simulink model "Modelling2018"  (R2018b)
settings: Solver=VariableStepAuto  StartTime=0.0  StopTime=50  FixedStep=1/16000  RelTol=1e-3
values from neighbouring files (symbols this model uses):
  A = [0 1 0 0 ... (first row only)    [ControllerToProject.m]
  B = [0 0 ... (first row only)    [ControllerToProject.m]
  b = 1    [ControllerToProject.m]    (also in Parameters.m)
  C = [1 0 0 0 ... (first row only)    [ControllerToProject.m]
  g = 9.81    [ControllerToProject.m]    (also in Parameters.m = 9.82)
  l = 0.36022    [ControllerToProject.m]    (also in Parameters.m = 0.35)
  mc = 0.9+0.1    (= 1)    [ControllerToProject.m]    (also in Parameters.m = 0.9)
  mp = 0.08887    [ControllerToProject.m]    (also in Parameters.m = 0.1)
undefined symbols (not defined in the file or in its folder): F, Fi, sigbuilder_block
libraries: simulink x9, simulink_extras x3
settings Model: Creator=Emil  LastModifiedBy=Emil
settings SolverCC: AlgebraicLoopSolver=LineSearch
settings DataIOCC: ReturnWorkspaceOutputs=on

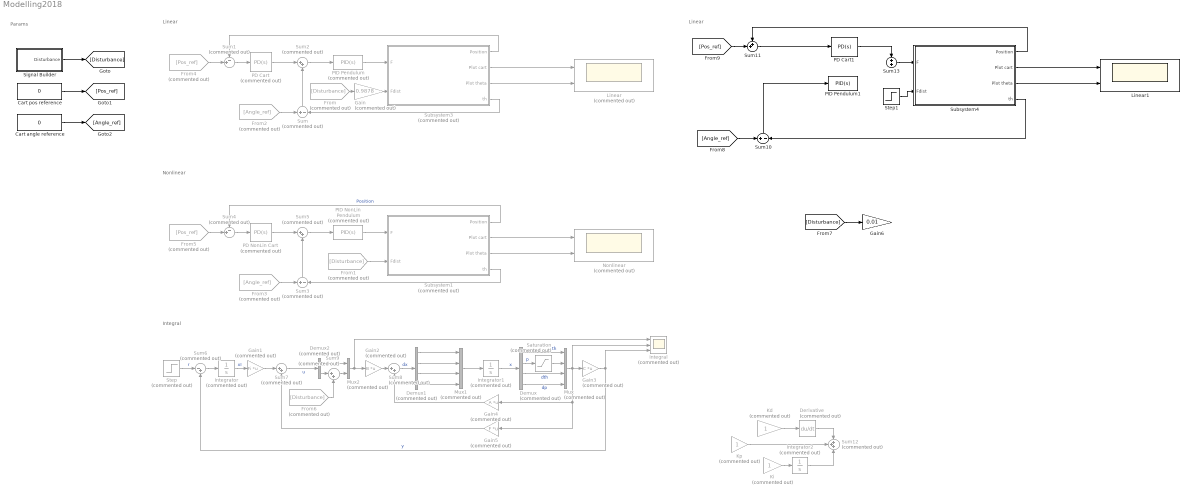
== system Modelling2018 ==
  note: Params
  note: Nonlinear
  note: Linear
  note: Integral
  note: Linear
  Cart angle reference : Constant  Value=0
  Cart pos reference : Constant  Value=0
  Demux : Demux  Commented=on
  Demux1 : Demux  Commented=on
  Demux2 : Demux  Commented=on  Outputs=2
  Derivative : Derivative  Commented=on
  From : From  Commented=on  GotoTag=Disturbance
  From1 : From  Commented=on  GotoTag=Disturbance
  From2 : From  Commented=on  GotoTag=Angle_ref
  From3 : From  Commented=on  GotoTag=Angle_ref
  From4 : From  Commented=on  GotoTag=Pos_ref
  From5 : From  Commented=on  GotoTag=Pos_ref
  From6 : From  Commented=on  GotoTag=Disturbance
  Gain : Gain  Commented=on  Gain=0.9878
  Gain1 : Gain  Commented=on  Gain=Fi  Multiplication=Matrix(K*u)
  Gain2 : Gain  Commented=on  Gain=B  Multiplication=Matrix(K*u)
  Gain3 : Gain  Commented=on  Gain=C  Multiplication=Matrix(K*u)
  Gain4 : Gain  Commented=on  Gain=A  Multiplication=Matrix(K*u)
  Gain5 : Gain  Commented=on  Gain=F  Multiplication=Matrix(K*u)
  Gain6 : Gain  Gain=0.01
  Integral : Scope  Commented=on  NumInputPorts=3
  Integrator : Integrator  Commented=on
  Integrator1 : Integrator  Commented=on
  Integrator2 : Integrator  Commented=on
  Kd : Gain  Commented=on
  Ki : Gain  Commented=on
  Kp : Gain  Commented=on
  Linear : Scope  Commented=on  NumInputPorts=2
  Linear1 : Scope  NumInputPorts=2
  Mux : Mux  Commented=on
  Mux1 : Mux  Commented=on
  Mux2 : Mux  Commented=on  Inputs=2
  Nonlinear : Scope  Commented=on  NumInputPorts=2
  PD Cart : simulink/Continuous/PID Controller  Commented=on  Controller=PD  Form=Ideal  TimeDomain=Continuous-time  SampleTime=-1  IntegratorMethod=Forward Euler  FilterMethod=Forward Euler  ControllerParametersSource=internal  P=1  I=0  D=0.017  UseFilter=on  N=100  TunerSelectOption=Transfer Function Based (PID Tuner App)  InitialConditionSource=internal  InitialConditionForIntegrator=0  InitialConditionForFilter=0  DifferentiatorICPrevScaledInput=0  ExternalReset=none  TrackingMode=off  Kt=1  LimitOutput=off  UpperSaturationLimit=inf  LowerSaturationLimit=-inf  LinearizeAsGain=on  AntiWindupMode=none  Kb=1  POutMin=[]  POutMax=[]  IOutMin=[]  IOutMax=[]  DOutMin=[]  DOutMax=[]  NOutMin=[]  NOutMax=[]  SumOutMin=[]  SumOutMax=[]  SaturationOutMin=[]  SaturationOutMax=[]  PParamMin=[]  PParamMax=[]  IParamMin=[]  IParamMax=[]  DParamMin=[]  DParamMax=[]  NParamMin=[]  NParamMax=[]  KbParamMin=[]  KbParamMax=[]  KtParamMin=[]  KtParamMax=[]  KbOutMin=[]  KbOutMax=[]  KtOutMin=[]  KtOutMax=[]  IntegratorOutMin=[]  IntegratorOutMax=[]  FilterOutMin=[]  FilterOutMax=[]  SumI1OutMin=[]  SumI1OutMax=[]  SumI2OutMin=[]  SumI2OutMax=[]  SumI3OutMin=[]  SumI3OutMax=[]  SumI4OutMin=[]  SumI4OutMax=[]  SumDOutMin=[]  SumDOutMax=[]  DifferentiatorOutMin=[]  DifferentiatorOutMax=[]  FilterDiffOutCoefMin=[]  FilterDiffOutCoefMax=[]  ReciprocalOutMin=[]  ReciprocalOutMax=[]  SumDenOutMin=[]  SumDenOutMax=[]  SumNumOutMin=[]  SumNumOutMax=[]  DivideOutMin=[]  DivideOutMax=[]  IntegratorContinuousStateAttributes=''  IntegratorStateMustResolveToSignalObject=off  IntegratorRTWStateStorageClass=Auto  FilterContinuousStateAttributes=''  FilterStateMustResolveToSignalObject=off  FilterRTWStateStorageClass=Auto  ParallelPVariant=Passthrough  IdealPVariant=InternalParameters  IVariant=Disabled  DVariant=InternalParameters  IntegratorVariant=Disabled  SatVariant=Disabled  AWVariant=Disabled  PCopyVariant=Disabled  TRVariant=Disabled  FdbkBlocksVariant=Forward  IdealPFdbkVariant=Disabled  SatFdbkVariant=Disabled  DerivativeFilterVariant=ContFilter  NVariant=InternalParameters  NCopyVariant=Disabled  FilterICVariant=InternalICsFilter  IntegratorICVariant=Disabled  ExternalResetVariant=Disabled  TRSumVariant=Passthrough  SumFdbkVariant=Disabled  SumVariant=Sum_PD
  PD Cart1 : simulink/Continuous/PID Controller  Controller=PD  Form=Parallel  TimeDomain=Continuous-time  SampleTime=-1  IntegratorMethod=Forward Euler  FilterMethod=Forward Euler  ControllerParametersSource=internal  P=1  I=1793804776.75566  D=0  UseFilter=on  N=100  TunerSelectOption=Transfer Function Based (PID Tuner App)  InitialConditionSource=internal  InitialConditionForIntegrator=0  InitialConditionForFilter=0  DifferentiatorICPrevScaledInput=0  ExternalReset=none  TrackingMode=off  Kt=1  LimitOutput=off  UpperSaturationLimit=50  LowerSaturationLimit=-50  LinearizeAsGain=on  AntiWindupMode=none  Kb=1  POutMin=[]  POutMax=[]  IOutMin=[]  IOutMax=[]  DOutMin=[]  DOutMax=[]  NOutMin=[]  NOutMax=[]  SumOutMin=[]  SumOutMax=[]  SaturationOutMin=[]  SaturationOutMax=[]  PParamMin=[]  PParamMax=[]  IParamMin=[]  IParamMax=[]  DParamMin=[]  DParamMax=[]  NParamMin=[]  NParamMax=[]  KbParamMin=[]  KbParamMax=[]  KtParamMin=[]  KtParamMax=[]  KbOutMin=[]  KbOutMax=[]  KtOutMin=[]  KtOutMax=[]  IntegratorOutMin=[]  IntegratorOutMax=[]  FilterOutMin=[]  FilterOutMax=[]  SumI1OutMin=[]  SumI1OutMax=[]  SumI2OutMin=[]  SumI2OutMax=[]  SumI3OutMin=[]  SumI3OutMax=[]  SumI4OutMin=[]  SumI4OutMax=[]  SumDOutMin=[]  SumDOutMax=[]  DifferentiatorOutMin=[]  DifferentiatorOutMax=[]  FilterDiffOutCoefMin=[]  FilterDiffOutCoefMax=[]  ReciprocalOutMin=[]  ReciprocalOutMax=[]  SumDenOutMin=[]  SumDenOutMax=[]  SumNumOutMin=[]  SumNumOutMax=[]  DivideOutMin=[]  DivideOutMax=[]  IntegratorContinuousStateAttributes=''  IntegratorStateMustResolveToSignalObject=off  IntegratorRTWStateStorageClass=Auto  FilterContinuousStateAttributes=''  FilterStateMustResolveToSignalObject=off  FilterRTWStateStorageClass=Auto  ParallelPVariant=InternalParameters  IdealPVariant=Disabled  IVariant=Disabled  DVariant=InternalParameters  IntegratorVariant=Disabled  SatVariant=Disabled  AWVariant=Disabled  PCopyVariant=Disabled  TRVariant=Disabled  FdbkBlocksVariant=Forward  IdealPFdbkVariant=Disabled  SatFdbkVariant=Disabled  DerivativeFilterVariant=ContFilter  NVariant=InternalParameters  NCopyVariant=Disabled  FilterICVariant=InternalICsFilter  IntegratorICVariant=Disabled  ExternalResetVariant=Disabled  TRSumVariant=Passthrough  SumFdbkVariant=Disabled  SumVariant=Sum_PD
  PD NonLin Cart : simulink/Continuous/PID Controller  Commented=on  Controller=PD  Form=Ideal  TimeDomain=Continuous-time  SampleTime=-1  IntegratorMethod=Forward Euler  FilterMethod=Forward Euler  ControllerParametersSource=internal  P=0.945  I=0  D=0.017  UseFilter=on  N=100  TunerSelectOption=Transfer Function Based (PID Tuner App)  InitialConditionSource=internal  InitialConditionForIntegrator=0  InitialConditionForFilter=0  DifferentiatorICPrevScaledInput=0  ExternalReset=none  TrackingMode=off  Kt=1  LimitOutput=off  UpperSaturationLimit=inf  LowerSaturationLimit=-inf  LinearizeAsGain=on  AntiWindupMode=none  Kb=1  POutMin=[]  POutMax=[]  IOutMin=[]  IOutMax=[]  DOutMin=[]  DOutMax=[]  NOutMin=[]  NOutMax=[]  SumOutMin=[]  SumOutMax=[]  SaturationOutMin=[]  SaturationOutMax=[]  PParamMin=[]  PParamMax=[]  IParamMin=[]  IParamMax=[]  DParamMin=[]  DParamMax=[]  NParamMin=[]  NParamMax=[]  KbParamMin=[]  KbParamMax=[]  KtParamMin=[]  KtParamMax=[]  KbOutMin=[]  KbOutMax=[]  KtOutMin=[]  KtOutMax=[]  IntegratorOutMin=[]  IntegratorOutMax=[]  FilterOutMin=[]  FilterOutMax=[]  SumI1OutMin=[]  SumI1OutMax=[]  SumI2OutMin=[]  SumI2OutMax=[]  SumI3OutMin=[]  SumI3OutMax=[]  SumI4OutMin=[]  SumI4OutMax=[]  SumDOutMin=[]  SumDOutMax=[]  DifferentiatorOutMin=[]  DifferentiatorOutMax=[]  FilterDiffOutCoefMin=[]  FilterDiffOutCoefMax=[]  ReciprocalOutMin=[]  ReciprocalOutMax=[]  SumDenOutMin=[]  SumDenOutMax=[]  SumNumOutMin=[]  SumNumOutMax=[]  DivideOutMin=[]  DivideOutMax=[]  IntegratorContinuousStateAttributes=''  IntegratorStateMustResolveToSignalObject=off  IntegratorRTWStateStorageClass=Auto  FilterContinuousStateAttributes=''  FilterStateMustResolveToSignalObject=off  FilterRTWStateStorageClass=Auto  ParallelPVariant=Passthrough  IdealPVariant=InternalParameters  IVariant=Disabled  DVariant=InternalParameters  IntegratorVariant=Disabled  SatVariant=Disabled  AWVariant=Disabled  PCopyVariant=Disabled  TRVariant=Disabled  FdbkBlocksVariant=Forward  IdealPFdbkVariant=Disabled  SatFdbkVariant=Disabled  DerivativeFilterVariant=ContFilter  NVariant=InternalParameters  NCopyVariant=Disabled  FilterICVariant=InternalICsFilter  IntegratorICVariant=Disabled  ExternalResetVariant=Disabled  TRSumVariant=Passthrough  SumFdbkVariant=Disabled  SumVariant=Sum_PD
  PID NonLin Pendulum : simulink/Continuous/PID Controller  Commented=on  Controller=PID  Form=Ideal  TimeDomain=Continuous-time  SampleTime=-1  IntegratorMethod=Forward Euler  FilterMethod=Forward Euler  ControllerParametersSource=internal  P=-500  I=55  D=5  UseFilter=on  N=500  TunerSelectOption=Transfer Function Based (PID Tuner App)  InitialConditionSource=internal  InitialConditionForIntegrator=0  InitialConditionForFilter=0  DifferentiatorICPrevScaledInput=0  ExternalReset=none  TrackingMode=off  Kt=1  LimitOutput=on  UpperSaturationLimit=50  LowerSaturationLimit=-50  LinearizeAsGain=on  AntiWindupMode=clamping  Kb=1  POutMin=[]  POutMax=[]  IOutMin=[]  IOutMax=[]  DOutMin=[]  DOutMax=[]  NOutMin=[]  NOutMax=[]  SumOutMin=[]  SumOutMax=[]  SaturationOutMin=[]  SaturationOutMax=[]  PParamMin=[]  PParamMax=[]  IParamMin=[]  IParamMax=[]  DParamMin=[]  DParamMax=[]  NParamMin=[]  NParamMax=[]  KbParamMin=[]  KbParamMax=[]  KtParamMin=[]  KtParamMax=[]  KbOutMin=[]  KbOutMax=[]  KtOutMin=[]  KtOutMax=[]  IntegratorOutMin=[]  IntegratorOutMax=[]  FilterOutMin=[]  FilterOutMax=[]  SumI1OutMin=[]  SumI1OutMax=[]  SumI2OutMin=[]  SumI2OutMax=[]  SumI3OutMin=[]  SumI3OutMax=[]  SumI4OutMin=[]  SumI4OutMax=[]  SumDOutMin=[]  SumDOutMax=[]  DifferentiatorOutMin=[]  DifferentiatorOutMax=[]  FilterDiffOutCoefMin=[]  FilterDiffOutCoefMax=[]  ReciprocalOutMin=[]  ReciprocalOutMax=[]  SumDenOutMin=[]  SumDenOutMax=[]  SumNumOutMin=[]  SumNumOutMax=[]  DivideOutMin=[]  DivideOutMax=[]  IntegratorContinuousStateAttributes=''  IntegratorStateMustResolveToSignalObject=off  IntegratorRTWStateStorageClass=Auto  FilterContinuousStateAttributes=''  FilterStateMustResolveToSignalObject=off  FilterRTWStateStorageClass=Auto  ParallelPVariant=Passthrough  IdealPVariant=InternalParameters  IVariant=InternalParameters  DVariant=InternalParameters  IntegratorVariant=Continuous  SatVariant=Enabled  AWVariant=ContClampingIdeal  PCopyVariant=InternalParamsIdeal  TRVariant=Disabled  FdbkBlocksVariant=Forward  IdealPFdbkVariant=Disabled  SatFdbkVariant=Disabled  DerivativeFilterVariant=ContFilter  NVariant=InternalParameters  NCopyVariant=Disabled  FilterICVariant=InternalICsFilter  IntegratorICVariant=InternalICs  ExternalResetVariant=Disabled  TRSumVariant=Passthrough  SumFdbkVariant=Disabled  SumVariant=Sum_PID
  PID Pendulum : simulink/Continuous/PID Controller  Commented=on  Controller=PID  Form=Ideal  TimeDomain=Continuous-time  SampleTime=-1  IntegratorMethod=Forward Euler  FilterMethod=Forward Euler  ControllerParametersSource=internal  P=-500  I=0.01  D=5  UseFilter=on  N=500  TunerSelectOption=Transfer Function Based (PID Tuner App)  InitialConditionSource=internal  InitialConditionForIntegrator=0  InitialConditionForFilter=0  DifferentiatorICPrevScaledInput=0  ExternalReset=none  TrackingMode=off  Kt=1  LimitOutput=on  UpperSaturationLimit=50  LowerSaturationLimit=-50  LinearizeAsGain=on  AntiWindupMode=clamping  Kb=1  POutMin=[]  POutMax=[]  IOutMin=[]  IOutMax=[]  DOutMin=[]  DOutMax=[]  NOutMin=[]  NOutMax=[]  SumOutMin=[]  SumOutMax=[]  SaturationOutMin=[]  SaturationOutMax=[]  PParamMin=[]  PParamMax=[]  IParamMin=[]  IParamMax=[]  DParamMin=[]  DParamMax=[]  NParamMin=[]  NParamMax=[]  KbParamMin=[]  KbParamMax=[]  KtParamMin=[]  KtParamMax=[]  KbOutMin=[]  KbOutMax=[]  KtOutMin=[]  KtOutMax=[]  IntegratorOutMin=[]  IntegratorOutMax=[]  FilterOutMin=[]  FilterOutMax=[]  SumI1OutMin=[]  SumI1OutMax=[]  SumI2OutMin=[]  SumI2OutMax=[]  SumI3OutMin=[]  SumI3OutMax=[]  SumI4OutMin=[]  SumI4OutMax=[]  SumDOutMin=[]  SumDOutMax=[]  DifferentiatorOutMin=[]  DifferentiatorOutMax=[]  FilterDiffOutCoefMin=[]  FilterDiffOutCoefMax=[]  ReciprocalOutMin=[]  ReciprocalOutMax=[]  SumDenOutMin=[]  SumDenOutMax=[]  SumNumOutMin=[]  SumNumOutMax=[]  DivideOutMin=[]  DivideOutMax=[]  IntegratorContinuousStateAttributes=''  IntegratorStateMustResolveToSignalObject=off  IntegratorRTWStateStorageClass=Auto  FilterContinuousStateAttributes=''  FilterStateMustResolveToSignalObject=off  FilterRTWStateStorageClass=Auto  ParallelPVariant=Passthrough  IdealPVariant=InternalParameters  IVariant=InternalParameters  DVariant=InternalParameters  IntegratorVariant=Continuous  SatVariant=Enabled  AWVariant=ContClampingIdeal  PCopyVariant=InternalParamsIdeal  TRVariant=Disabled  FdbkBlocksVariant=Forward  IdealPFdbkVariant=Disabled  SatFdbkVariant=Disabled  DerivativeFilterVariant=ContFilter  NVariant=InternalParameters  NCopyVariant=Disabled  FilterICVariant=InternalICsFilter  IntegratorICVariant=InternalICs  ExternalResetVariant=Disabled  TRSumVariant=Passthrough  SumFdbkVariant=Disabled  SumVariant=Sum_PID
  PID Pendulum1 : simulink/Continuous/PID Controller  Controller=PID  Form=Parallel  TimeDomain=Continuous-time  SampleTime=-1  IntegratorMethod=Forward Euler  FilterMethod=Forward Euler  ControllerParametersSource=internal  P=1  I=1  D=1  UseFilter=on  N=100  TunerSelectOption=Transfer Function Based (PID Tuner App)  InitialConditionSource=internal  InitialConditionForIntegrator=0  InitialConditionForFilter=0  DifferentiatorICPrevScaledInput=0  ExternalReset=none  TrackingMode=off  Kt=1  LimitOutput=on  UpperSaturationLimit=50  LowerSaturationLimit=-50  LinearizeAsGain=on  AntiWindupMode=clamping  Kb=1  POutMin=[]  POutMax=[]  IOutMin=[]  IOutMax=[]  DOutMin=[]  DOutMax=[]  NOutMin=[]  NOutMax=[]  SumOutMin=[]  SumOutMax=[]  SaturationOutMin=[]  SaturationOutMax=[]  PParamMin=[]  PParamMax=[]  IParamMin=[]  IParamMax=[]  DParamMin=[]  DParamMax=[]  NParamMin=[]  NParamMax=[]  KbParamMin=[]  KbParamMax=[]  KtParamMin=[]  KtParamMax=[]  KbOutMin=[]  KbOutMax=[]  KtOutMin=[]  KtOutMax=[]  IntegratorOutMin=[]  IntegratorOutMax=[]  FilterOutMin=[]  FilterOutMax=[]  SumI1OutMin=[]  SumI1OutMax=[]  SumI2OutMin=[]  SumI2OutMax=[]  SumI3OutMin=[]  SumI3OutMax=[]  SumI4OutMin=[]  SumI4OutMax=[]  SumDOutMin=[]  SumDOutMax=[]  DifferentiatorOutMin=[]  DifferentiatorOutMax=[]  FilterDiffOutCoefMin=[]  FilterDiffOutCoefMax=[]  ReciprocalOutMin=[]  ReciprocalOutMax=[]  SumDenOutMin=[]  SumDenOutMax=[]  SumNumOutMin=[]  SumNumOutMax=[]  DivideOutMin=[]  DivideOutMax=[]  IntegratorContinuousStateAttributes=''  IntegratorStateMustResolveToSignalObject=off  IntegratorRTWStateStorageClass=Auto  FilterContinuousStateAttributes=''  FilterStateMustResolveToSignalObject=off  FilterRTWStateStorageClass=Auto  ParallelPVariant=InternalParameters  IdealPVariant=Disabled  IVariant=InternalParameters  DVariant=InternalParameters  IntegratorVariant=Continuous  SatVariant=Enabled  AWVariant=ContClampingParallel  PCopyVariant=Disabled  TRVariant=Disabled  FdbkBlocksVariant=Forward  IdealPFdbkVariant=Disabled  SatFdbkVariant=Disabled  DerivativeFilterVariant=ContFilter  NVariant=InternalParameters  NCopyVariant=Disabled  FilterICVariant=InternalICsFilter  IntegratorICVariant=InternalICs  ExternalResetVariant=Disabled  TRSumVariant=Passthrough  SumFdbkVariant=Disabled  SumVariant=Sum_PID
  Saturation : Saturate  Commented=on  UpperLimit=0.8  LowerLimit=-0.8
  Signal Builder : Subsystem  Tag=STV Subsys  LoadFcn=sigbuilder_block('load');  StartFcn=sigbuilder_block('start');  StopFcn=sigbuilder_block('stop');  ClipboardFcn=sigbuilder_block('clipboard');  mask(Sigbuilder block){tuvar=[0:10]}
      mask help: Simulink:masks:SigbuilderBlock_MD
      mask init:
      | if ~strcmp(get_param(bdroot(gcbh),'SimulationStatus'),'stopped') tuvar = sigbuilder_block('maskInit'); end
      settings: CopyFcn=sigbuilder_block('copy');  DeleteFcn=sigbuilder_block('delete');  ModelCloseFcn=sigbuilder_block('modelClose');  PreSaveFcn=sigbuilder_block('preSave');  PauseFcn=sigbuilder_block('pause');  ContinueFcn=sigbuilder_block('continue');  NameChangeFcn=sigbuilder_block('namechange');  OpenFcn=sigbuilder_block('open',[3.75 670.5 818.25 342 ]);  CloseFcn=sigbuilder_block('close');
      mask Display: plot(0, 0, 100, 100,[2, 2, 32, 32, 2], [68, 8, 8, 68, 68],[32, 2], [38, 38], [32, 19, 2],[53, 60, 44], [32, 17, 17, 2],[16, 16, 31, 31]);txt = getActiveGroup(gcbh);text(2, 100, txt,'verticalAlignment', 'top');
  Step : Step  Commented=on  Time=0  Before=[0, 0]  After=[0, 0.2]  SampleTime=0
  Step1 : Step  Before=0.1  After=0  SampleTime=0
  Subsystem1 : Subsystem  Commented=on
      mask Display: image('System.png'); % Use "Edit Image" on toolstrip to change.
  Subsystem3 : Subsystem  Commented=on
      mask Display: image('System.png'); % Use "Edit Image" on toolstrip to change.
  Subsystem4 : Subsystem
      mask Display: image('System.png'); % Use "Edit Image" on toolstrip to change.
  Sum : Sum  Commented=on  Inputs=+-
  Sum1 : Sum  Commented=on  Inputs=-+|
  Sum10 : Sum  Inputs=+-
  Sum11 : Sum  Inputs=++|
  Sum12 : Sum  Commented=on  Inputs=+++
  Sum13 : Sum
  Sum{2,5,7..9} (5 alike) : Sum  Commented=on  Inputs=|++
  Sum3 : Sum  Commented=on  Inputs=+-
  Sum4 : Sum  Commented=on  Inputs=-+|
  Sum6 : Sum  Commented=on  Inputs=|-+
  wires:
  Subsystem3/1(Position) -> Sum1/1
  Subsystem3/4(th) -> Sum/2
  From2/1 -> Sum/1
  From4/1 -> Sum1/2
  Sum/1 -> Sum2/2
  Sum2/1 -> PID Pendulum/1
  Sum1/1 -> PD Cart/1
  PD Cart/1 -> Sum2/1
  From5/1 -> Sum4/2
  From3/1 -> Sum3/1
  Sum3/1 -> Sum5/2
  Subsystem1/1(Position) -> Sum4/1  "Position"
  Subsystem1/4(th) -> Sum3/2
  PID Pendulum/1 -> Subsystem3/1(F)
  Subsystem1/3(Plot theta) -> Nonlinear/2
  PID NonLin Pendulum/1 -> Subsystem1/1(F)
  Sum5/1 -> PID NonLin Pendulum/1
  Sum4/1 -> PD NonLin Cart/1
  PD NonLin Cart/1 -> Sum5/1
  Signal Builder/1(Disturbance) -> [Disturbance]
  From1/1 -> Subsystem1/2(Fdist)
  Cart pos reference/1 -> [Pos_ref]
  Cart angle reference/1 -> [Angle_ref]
  Subsystem1/2(Plot cart) -> Nonlinear/1
  Subsystem3/2(Plot cart) -> Linear/1
  Subsystem3/3(Plot theta) -> Linear/2
  From/1 -> Gain/1
  Gain/1 -> Subsystem3/2(Fdist)
  Sum6/1 -> Integrator/1
  Gain3/1 -> Integral/3, Sum6/2  "y"
  Gain1/1 -> Sum7/1
  Gain2/1 -> Sum8/1
  Gain5/1 -> Sum7/2
  Step/1 -> Sum6/1  "r"
  Gain4/1 -> Sum8/2
  Integrator1/1 -> Demux/1  "x"
  Demux/2 -> Saturation/1  "p"
  Saturation/1 -> Mux/2
  Demux/3 -> Mux/3  "dth"
  Demux/4 -> Mux/4  "dp"
  Mux/1 -> Integral/2, Gain5/1, Gain4/1, Gain3/1
  Demux1/4 -> Mux1/4
  Demux1/3 -> Mux1/3
  Sum8/1 -> Demux1/1  "dx"
  Mux1/1 -> Integrator1/1
  Demux1/2 -> Mux1/2
  Demux1/1 -> Mux1/1
  Demux/1 -> Mux/1  "th"
  Integrator/1 -> Gain1/1  "xI"
  Sum9/1 -> Mux2/2
  Sum7/1 -> Demux2/1  "u"
  Mux2/1 -> Integral/1, Gain2/1
  Demux2/1 -> Mux2/1
  Demux2/2 -> Sum9/1
  From6/1 -> Sum9/2
  [Angle_ref] -> Sum10/1
  Subsystem4/4(th) -> Sum10/2
  Subsystem4/1(Position) -> Sum11/1
  Subsystem4/3(Plot theta) -> Linear1/2
  Subsystem4/2(Plot cart) -> Linear1/1
  [Pos_ref] -> Sum11/2
  Sum13/1 -> Subsystem4/1(F)
  ? -> Ki/1, Kd/1, Kp/1
  Ki/1 -> Integrator2/1
  Integrator2/1 -> Sum12/3
  Derivative/1 -> Sum12/1
  Kd/1 -> Derivative/1
  Kp/1 -> Sum12/2
  PD Cart1/1 -> Sum13/1
  Sum10/1 -> PID Pendulum1/1
  Sum11/1 -> PD Cart1/1
  [Disturbance] -> Gain6/1
  Step1/1 -> Subsystem4/2(Fdist)

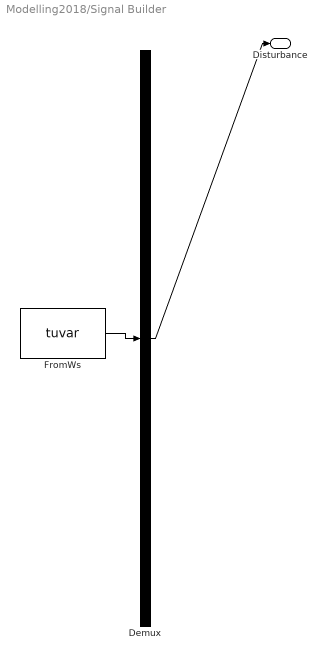
== system Modelling2018/Signal Builder ==
  Demux : Demux  Tag=STV Demux  Outputs=1
      settings: DisplayOption=none
  FromWs : FromWorkspace  Tag=STV FromWs  VariableName=tuvar
      SigBuilderData=|
      | common.afterFinalStr = 'Extrapolate'
      | common.sampleTime = 0
      | dataSet.timeRange = [0 10]
      | dataSet.name = 'Group 1'
      | sbobj.Groups.Name = 'Group 1'
      | sbobj.Groups.Signals.Name = 'Disturbance'
      | sbobj.Groups.Signals.XData = [0 0.25 0.5 0.75 1 1.25 1.5 1.75 2 2.25 2.5 2.75 3 3.25 3.5 3.75 4 4.25 4.5 4.75 5 5.25 5.5 5.75 6 6.25 6.5 6.75 7 7.25 7.5 7.75 8 8.25 8.5 8.75 9 9.25 9.5 9.75 10]
      | sbobj.Groups.Signals.YData = [0 0 0 0 0 0 0 0 0 0 0 -2.77555756156e-17 -0.002 0.063 0.002 -0.03 -0.05 -0.05 0.01 -0.146 0.16 0.08 0.1 0.089 0.193 0.06 0.02 -2.7756e-18 -0.022 -0.034 -0.099 -0.084 -0.01 -0.02 -0.051 -0.045 0.02 0.02 0.176 -2.7756e-18 -2.77555756156e-17]
  Disturbance : Outport  Tag=STV Outport
  wires:
  FromWs/1 -> Demux/1
  Demux/1 -> Disturbance/1

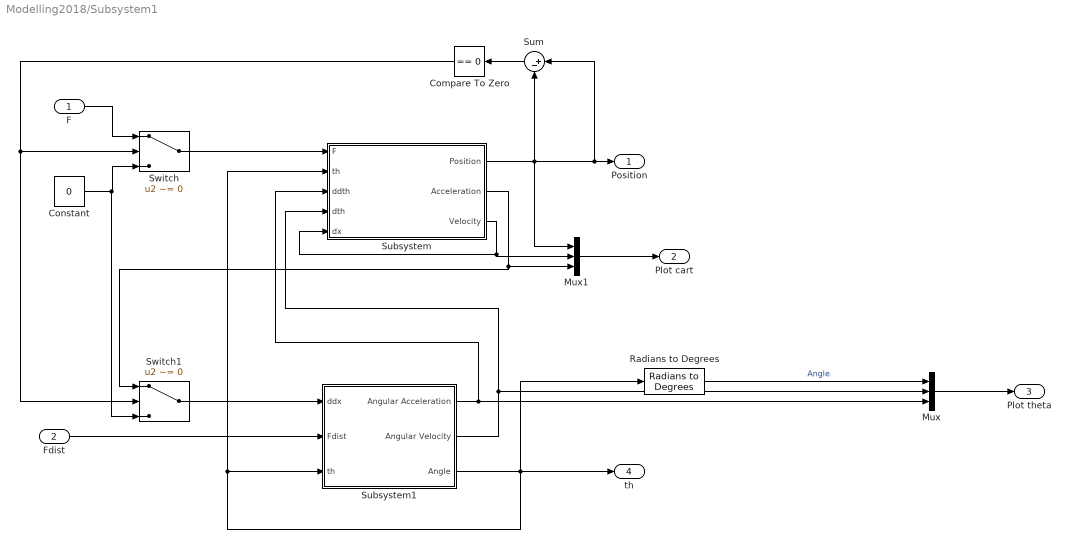
== system Modelling2018/Subsystem1 ==
  F : Inport
  Fdist : Inport  Port=2
  Compare To Zero : simulink/Logic and Bit Operations/Compare To Zero  relop===  OutDataTypeStr=boolean
  Constant : Constant  Value=0
  Mux : Mux  Inputs=3
  Mux1 : Mux  Inputs=3
  Radians to Degrees : simulink_extras/Transformations/Radians to Degrees
  Subsystem : Subsystem
      mask Display: image('Cart.png'); % Use "Edit Image" on toolstrip to change.
  Subsystem1 : Subsystem
      mask Display: image('Pendulum.png'); % Use "Edit Image" on toolstrip to change.
  Sum : Sum  Inputs=|+-
  Switch : Switch  Criteria=u2 ~= 0
  Switch1 : Switch  Criteria=u2 ~= 0
  Position : Outport
  Plot cart : Outport  Port=2
  Plot theta : Outport  Port=3
  th : Outport  Port=4
  wires:
  Fdist/1 -> Subsystem1/2(Fdist)
  Subsystem/3(Velocity) -> Mux1/2, Subsystem/5(dx)
  Subsystem1/3(Angle) -> th/1, Subsystem/2(th), Subsystem1/3(th), Radians to Degrees/1
  Subsystem1/2(Angular Velocity) -> Subsystem/4(dth), Mux/2
  Subsystem1/1(Angular Acceleration) -> Subsystem/3(ddth), Mux/3
  Sum/1 -> Compare To Zero/1
  Subsystem/1(Position) -> Sum/1, Position/1, Mux1/1, Sum/2
  F/1 -> Switch/1
  Constant/1 -> Switch1/3, Switch/3
  Compare To Zero/1 -> Switch1/2, Switch/2
  Switch/1 -> Subsystem/1(F)
  Switch1/1 -> Subsystem1/1(ddx)
  Subsystem/2(Acceleration) -> Switch1/1, Mux1/3
  Mux/1 -> Plot theta/1
  Mux1/1 -> Plot cart/1
  Radians to Degrees/1 -> Mux/1  "Angle"

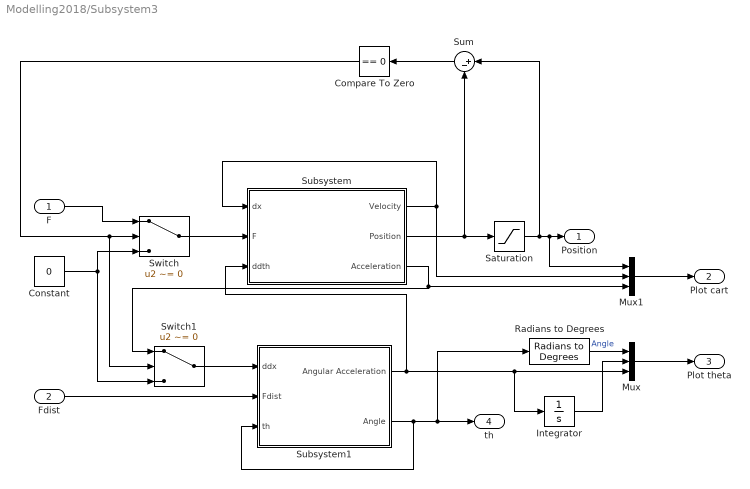
== system Modelling2018/Subsystem3 ==
  F : Inport
  Fdist : Inport  Port=2
  Compare To Zero : simulink/Logic and Bit Operations/Compare To Zero  relop===  OutDataTypeStr=boolean
  Constant : Constant  Value=0
  Integrator : Integrator
  Mux : Mux  Inputs=3
  Mux1 : Mux  Inputs=3
  Radians to Degrees : simulink_extras/Transformations/Radians to Degrees
  Saturation : Saturate  UpperLimit=0.8  LowerLimit=-0.8
  Subsystem : Subsystem
      mask Display: image('Cart.png'); % Use "Edit Image" on toolstrip to change.
  Subsystem1 : Subsystem
      mask Display: image('Pendulum.png'); % Use "Edit Image" on toolstrip to change.
  Sum : Sum  Inputs=|+-
  Switch : Switch  Criteria=u2 ~= 0
  Switch1 : Switch  Criteria=u2 ~= 0
  Position : Outport
  Plot cart : Outport  Port=2
  Plot theta : Outport  Port=3
  th : Outport  Port=4
  wires:
  F/1 -> Switch/1
  Fdist/1 -> Subsystem1/2(Fdist)
  Subsystem/2(Position) -> Saturation/1, Sum/2
  Sum/1 -> Compare To Zero/1
  Constant/1 -> Switch1/3, Switch/3
  Compare To Zero/1 -> Switch1/2, Switch/2
  Switch/1 -> Subsystem/2(F)
  Switch1/1 -> Subsystem1/1(ddx)
  Subsystem1/2(Angle) -> Radians to Degrees/1, th/1, Subsystem1/3(th)
  Subsystem1/1(Angular Acceleration) -> Integrator/1, Mux/3, Subsystem/3(ddth)
  Mux1/1 -> Plot cart/1
  Subsystem/3(Acceleration) -> Switch1/1, Mux1/3
  Integrator/1 -> Mux/2
  Subsystem/1(Velocity) -> Mux1/2, Subsystem/1(dx)
  Saturation/1 -> Sum/1, Mux1/1, Position/1
  Mux/1 -> Plot theta/1
  Radians to Degrees/1 -> Mux/1  "Angle"

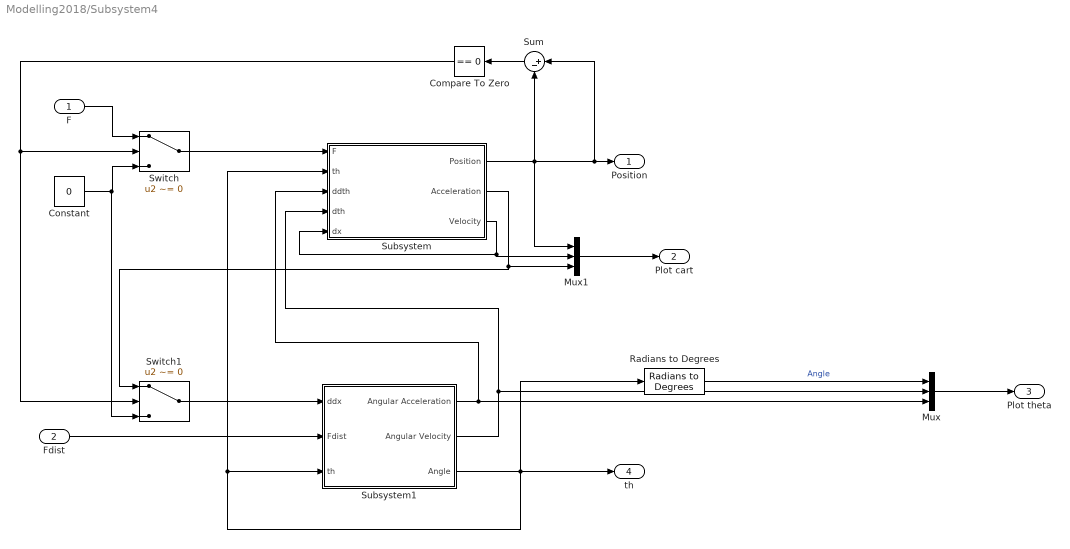
== system Modelling2018/Subsystem4 ==
  F : Inport
  Fdist : Inport  Port=2
  Compare To Zero : simulink/Logic and Bit Operations/Compare To Zero  relop===  OutDataTypeStr=boolean
  Constant : Constant  Value=0
  Mux : Mux  Inputs=3
  Mux1 : Mux  Inputs=3
  Radians to Degrees : simulink_extras/Transformations/Radians to Degrees
  Subsystem : Subsystem
      mask Display: image('Cart.png'); % Use "Edit Image" on toolstrip to change.
  Subsystem1 : Subsystem
      mask Display: image('Pendulum.png'); % Use "Edit Image" on toolstrip to change.
  Sum : Sum  Inputs=|+-
  Switch : Switch  Criteria=u2 ~= 0
  Switch1 : Switch  Criteria=u2 ~= 0
  Position : Outport
  Plot cart : Outport  Port=2
  Plot theta : Outport  Port=3
  th : Outport  Port=4
  wires:
  Fdist/1 -> Subsystem1/2(Fdist)
  Subsystem/3(Velocity) -> Mux1/2, Subsystem/5(dx)
  Subsystem1/3(Angle) -> th/1, Subsystem/2(th), Subsystem1/3(th), Radians to Degrees/1
  Subsystem1/2(Angular Velocity) -> Subsystem/4(dth), Mux/2
  Subsystem1/1(Angular Acceleration) -> Subsystem/3(ddth), Mux/3
  Sum/1 -> Compare To Zero/1
  Subsystem/1(Position) -> Sum/1, Position/1, Mux1/1, Sum/2
  F/1 -> Switch/1
  Constant/1 -> Switch1/3, Switch/3
  Compare To Zero/1 -> Switch1/2, Switch/2
  Switch/1 -> Subsystem/1(F)
  Switch1/1 -> Subsystem1/1(ddx)
  Subsystem/2(Acceleration) -> Switch1/1, Mux1/3
  Mux/1 -> Plot theta/1
  Mux1/1 -> Plot cart/1
  Radians to Degrees/1 -> Mux/1  "Angle"

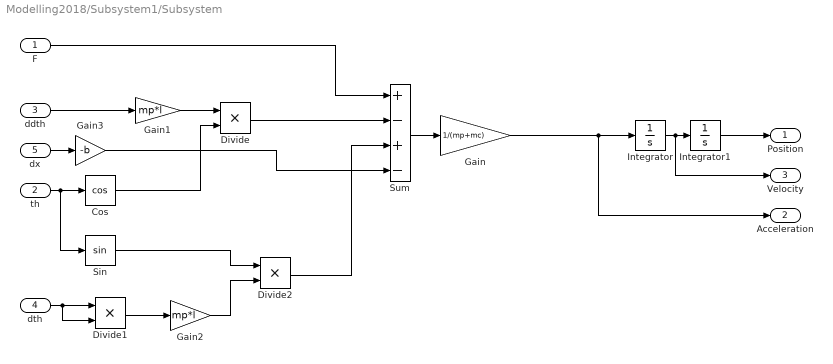
== system Modelling2018/Subsystem1/Subsystem ==
  F : Inport
  th : Inport  Port=2
  ddth : Inport  Port=3
  dth : Inport  Port=4
  dx : Inport  Port=5
  Cos : Trigonometry  Operator=cos
  Divide : Product  Inputs=**
  Divide1 : Product  Inputs=**
  Divide2 : Product  Inputs=**
  Gain : Gain  Gain=1/(mp+mc)
  Gain1 : Gain  Gain=mp*l
  Gain2 : Gain  Gain=mp*l
  Gain3 : Gain  Gain=-b
  Integrator : Integrator
  Integrator1 : Integrator
  Sin : Trigonometry
  Sum : Sum  Inputs=+-+-
  Position : Outport
  Acceleration : Outport  Port=2
  Velocity : Outport  Port=3
  wires:
  Sum/1 -> Gain/1
  th/1 -> Sin/1, Cos/1
  Integrator/1 -> Velocity/1, Integrator1/1
  Integrator1/1 -> Position/1
  ddth/1 -> Gain1/1
  Gain1/1 -> Divide/1
  Cos/1 -> Divide/2
  dth/1 -> Divide1/2, Divide1/1
  Divide1/1 -> Gain2/1
  Gain2/1 -> Divide2/2
  Sin/1 -> Divide2/1
  F/1 -> Sum/1
  Divide/1 -> Sum/2
  Divide2/1 -> Sum/3
  dx/1 -> Gain3/1
  Gain/1 -> Acceleration/1, Integrator/1
  Gain3/1 -> Sum/4

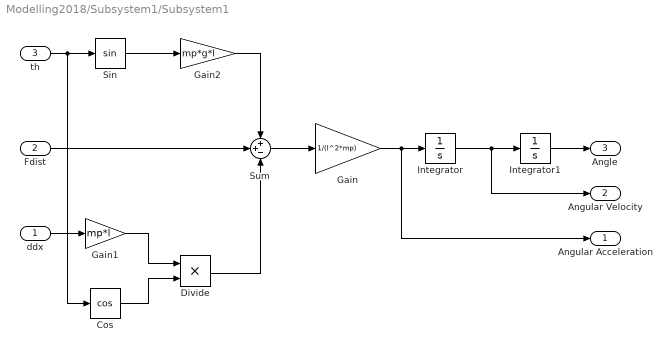
== system Modelling2018/Subsystem1/Subsystem1 ==
  ddx : Inport
  Fdist : Inport  Port=2
  th : Inport  Port=3
  Cos : Trigonometry  Operator=cos
  Divide : Product  Inputs=**
  Gain : Gain  Gain=1/(l^2*mp)
  Gain1 : Gain  Gain=mp*l
  Gain2 : Gain  Gain=mp*g*l
  Integrator : Integrator
  Integrator1 : Integrator
  Sin : Trigonometry
  Sum : Sum  Inputs=++-
  Angular Acceleration : Outport
  Angular Velocity : Outport  Port=2
  Angle : Outport  Port=3
  wires:
  Integrator/1 -> Angular Velocity/1, Integrator1/1
  Integrator1/1 -> Angle/1
  Gain/1 -> Angular Acceleration/1, Integrator/1
  Sum/1 -> Gain/1
  Fdist/1 -> Sum/2
  ddx/1 -> Gain1/1
  th/1 -> Sin/1, Cos/1
  Gain1/1 -> Divide/1
  Cos/1 -> Divide/2
  Divide/1 -> Sum/3
  Sin/1 -> Gain2/1
  Gain2/1 -> Sum/1

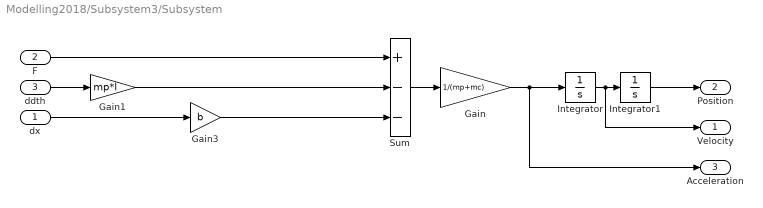
== system Modelling2018/Subsystem3/Subsystem ==
  dx : Inport
  F : Inport  Port=2
  ddth : Inport  Port=3
  Gain : Gain  Gain=1/(mp+mc)
  Gain1 : Gain  Gain=mp*l
  Gain3 : Gain  Gain=b
  Integrator : Integrator
  Integrator1 : Integrator
  Sum : Sum  Inputs=+--
  Velocity : Outport
  Position : Outport  Port=2
  Acceleration : Outport  Port=3
  wires:
  Sum/1 -> Gain/1
  Gain/1 -> Integrator/1, Acceleration/1
  Integrator/1 -> Velocity/1, Integrator1/1
  Integrator1/1 -> Position/1
  ddth/1 -> Gain1/1
  F/1 -> Sum/1
  Gain1/1 -> Sum/2
  dx/1 -> Gain3/1
  Gain3/1 -> Sum/3

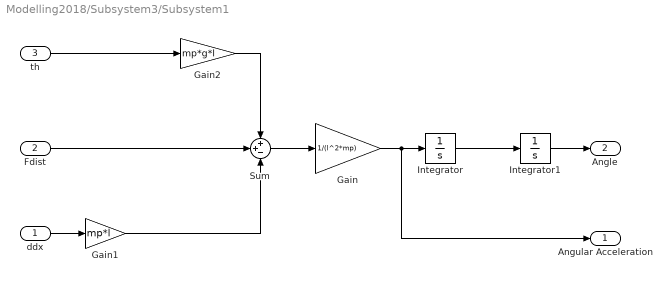
== system Modelling2018/Subsystem3/Subsystem1 ==
  ddx : Inport
  Fdist : Inport  Port=2
  th : Inport  Port=3
  Gain : Gain  Gain=1/(l^2*mp)
  Gain1 : Gain  Gain=mp*l
  Gain2 : Gain  Gain=mp*g*l
  Integrator : Integrator
  Integrator1 : Integrator
  Sum : Sum  Inputs=++-
  Angular Acceleration : Outport
  Angle : Outport  Port=2
  wires:
  Integrator/1 -> Integrator1/1
  Integrator1/1 -> Angle/1
  Gain/1 -> Angular Acceleration/1, Integrator/1
  Sum/1 -> Gain/1
  Fdist/1 -> Sum/2
  ddx/1 -> Gain1/1
  Gain1/1 -> Sum/3
  th/1 -> Gain2/1
  Gain2/1 -> Sum/1

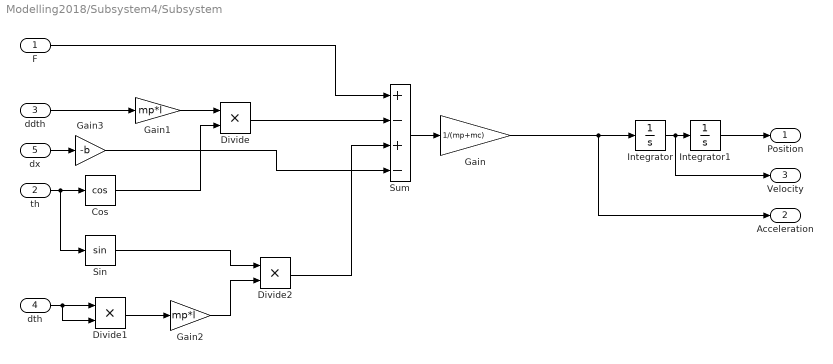
== system Modelling2018/Subsystem4/Subsystem ==
  F : Inport
  th : Inport  Port=2
  ddth : Inport  Port=3
  dth : Inport  Port=4
  dx : Inport  Port=5
  Cos : Trigonometry  Operator=cos
  Divide : Product  Inputs=**
  Divide1 : Product  Inputs=**
  Divide2 : Product  Inputs=**
  Gain : Gain  Gain=1/(mp+mc)
  Gain1 : Gain  Gain=mp*l
  Gain2 : Gain  Gain=mp*l
  Gain3 : Gain  Gain=-b
  Integrator : Integrator
  Integrator1 : Integrator
  Sin : Trigonometry
  Sum : Sum  Inputs=+-+-
  Position : Outport
  Acceleration : Outport  Port=2
  Velocity : Outport  Port=3
  wires:
  Sum/1 -> Gain/1
  th/1 -> Sin/1, Cos/1
  Integrator/1 -> Velocity/1, Integrator1/1
  Integrator1/1 -> Position/1
  ddth/1 -> Gain1/1
  Gain1/1 -> Divide/1
  Cos/1 -> Divide/2
  dth/1 -> Divide1/2, Divide1/1
  Divide1/1 -> Gain2/1
  Gain2/1 -> Divide2/2
  Sin/1 -> Divide2/1
  F/1 -> Sum/1
  Divide/1 -> Sum/2
  Divide2/1 -> Sum/3
  dx/1 -> Gain3/1
  Gain/1 -> Acceleration/1, Integrator/1
  Gain3/1 -> Sum/4

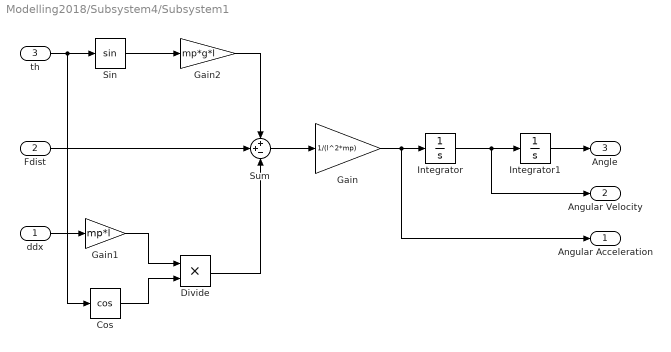
== system Modelling2018/Subsystem4/Subsystem1 ==
  ddx : Inport
  Fdist : Inport  Port=2
  th : Inport  Port=3
  Cos : Trigonometry  Operator=cos
  Divide : Product  Inputs=**
  Gain : Gain  Gain=1/(l^2*mp)
  Gain1 : Gain  Gain=mp*l
  Gain2 : Gain  Gain=mp*g*l
  Integrator : Integrator
  Integrator1 : Integrator
  Sin : Trigonometry
  Sum : Sum  Inputs=++-
  Angular Acceleration : Outport
  Angular Velocity : Outport  Port=2
  Angle : Outport  Port=3
  wires:
  Integrator/1 -> Angular Velocity/1, Integrator1/1
  Integrator1/1 -> Angle/1
  Gain/1 -> Angular Acceleration/1, Integrator/1
  Sum/1 -> Gain/1
  Fdist/1 -> Sum/2
  ddx/1 -> Gain1/1
  th/1 -> Sin/1, Cos/1
  Gain1/1 -> Divide/1
  Cos/1 -> Divide/2
  Divide/1 -> Sum/3
  Sin/1 -> Gain2/1
  Gain2/1 -> Sum/1
